simulink model "StopMotors"  (Simulink 7.3)
settings: Solver=FixedStepDiscrete  StartTime=0.0  StopTime=inf  FixedStep=1  RelTol=1e-3
settings Model: Creator=gclayton  LastModifiedBy=wildcat
settings RTWCC: SystemTargetFile=rlnx.tlc  GenCodeOnly=on  TemplateMakefile=rlnx_ubuntu.tmf  Description=Linux Real-Time Target  ProcessScript=rlnx_make_rtw_hook
settings CodeAppCC: GenerateComments=off  SimulinkBlockComments=off
settings STFCustomTargetCC: ModelReferenceCompliant=off  MatFileLogging=on  SystemTargetFile=rlnx.tlc
settings GRTTargetCC: ModelReferenceCompliant=off  ParMdlRefBuildCompliant=off  CompOptLevelCompliant=off
settings CustomProperty: DataType=string  Value=/matlab_includes/libfreenect/build/lib/libfreenect.so -lm -ldl
settings EnumStrPairs: String=PC

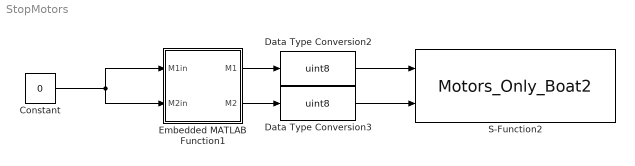
== system StopMotors ==
  Constant : Constant  Value=0  OutDataType=fixdt(1, 16)  OutScaling=2^0
  Data Type Conversion2 : DataTypeConversion  OutDataTypeMode=uint8  OutDataType=fixdt(1, 16)  OutScaling=2^0  OutDataTypeStr=uint8
  Data Type Conversion3 : DataTypeConversion  OutDataTypeMode=uint8  OutDataType=fixdt(1, 16)  OutScaling=2^0  OutDataTypeStr=uint8
  Embedded MATLAB Function1 : Stateflow chart
  S-Function2 : S-Function  FunctionName=Motors_Only_Boat2  EnableBusSupport=off
  wires:
  Embedded MATLAB Function1/1(M1) -> Data Type Conversion2/1
  Embedded MATLAB Function1/2(M2) -> Data Type Conversion3/1
  Data Type Conversion2/1 -> S-Function2/1
  Data Type Conversion3/1 -> S-Function2/2
  Constant/1 -> Embedded MATLAB Function1/1(M1in), Embedded MATLAB Function1/2(M2in)

== matlab function Embedded MATLAB Function1 ==
  data: M1in input double; M1 output double; M2in input double; M2 output double
function [M1, M2] = MotorPackets(M1in, M2in)
%#eml

M1 = 0;
M2 = 1;

if M1in <= 0
    M1 = M1+2;
end

if M2in <= 0
    M2 = M2+2;
end

M1 = M1 + round(abs(M1in)/15)*4;
M2 = M2 + round(abs(M2in)/15)*4;
